simulink model "baroreflex"  (Simulink 6.6)
settings: Solver=ode45  StartTime=0.0  StopTime=100  RelTol=1e-3
undefined symbols (not defined in the file or in its folder): sigbuilder_block
settings Model: Creator=niumi  LastModifiedBy=mxkana
settings DebuggingCC: MultiTaskDSMMsg=warning  MultiTaskCondExecSysMsg=none  StrictBusMsg=None
settings RTWCC: IncludeERTFirstTime=on

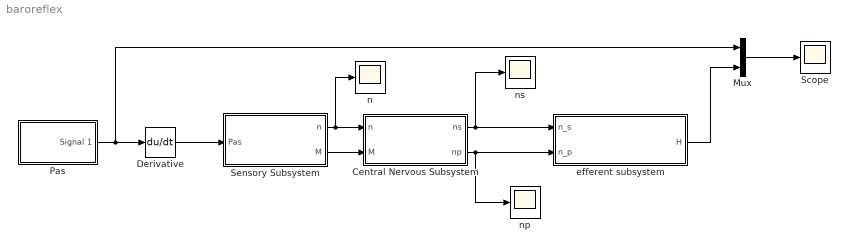
== system baroreflex ==
  Central Nervous Subsystem : Subsystem
  Derivative : Derivative
  Mux : Mux  Inputs=2
  Pas : Subsystem  Tag=STV Subsys  LoadFcn=sigbuilder_block('load');  StartFcn=sigbuilder_block('start');  StopFcn=sigbuilder_block('stop');  ClipboardFcn=sigbuilder_block('clipboard');  mask(Sigbuilder block){}
      mask help: Sigbuilder GUI
      mask init:
      | if ~strcmp(get_param(bdroot(gcbh),'SimulationStatus'),'stopped') tuvar = sigbuilder_block('maskInit'); end
      settings: CopyFcn=sigbuilder_block('copy');  DeleteFcn=sigbuilder_block('delete');  ModelCloseFcn=sigbuilder_block('modelClose');  PreSaveFcn=sigbuilder_block('preSave');  NameChangeFcn=sigbuilder_block('namechange');  OpenFcn=sigbuilder_block('open',[79.5 60.75 747 469.5 ]);  CloseFcn=sigbuilder_block('close');
      mask Display: plot(0,0,100,100,[10,10,40,40,10],[80,20,20,80,80],[40,10],[50,50], [40,27,10],[65,72,56],[40,25,25,10],[28,28,43,43]);
  Scope : Scope
      settings: YMin=0  YMax=100
  Sensory Subsystem : Subsystem
  "efferent subsystem " : Subsystem  TreatAsAtomicUnit=on
  n : Scope
      settings: YMin=0  YMax=100
  np : Scope
      settings: YMin=0  YMax=100  SaveName=ScopeData3
  ns : Scope
      settings: YMin=0  YMax=100  SaveName=ScopeData2
  wires:
  Sensory Subsystem/1(n) -> Central Nervous Subsystem/1(n), n/1
  Central Nervous Subsystem/1(ns) -> "efferent subsystem "/1(n_s), ns/1
  Central Nervous Subsystem/2(np) -> "efferent subsystem "/2(n_p), np/1
  Derivative/1 -> Sensory Subsystem/1(Pas)
  Pas/1(Signal 1) -> Derivative/1, Mux/1
  "efferent subsystem "/1(H) -> Mux/2
  Mux/1 -> Scope/1
  Sensory Subsystem/2(M) -> Central Nervous Subsystem/2(M)

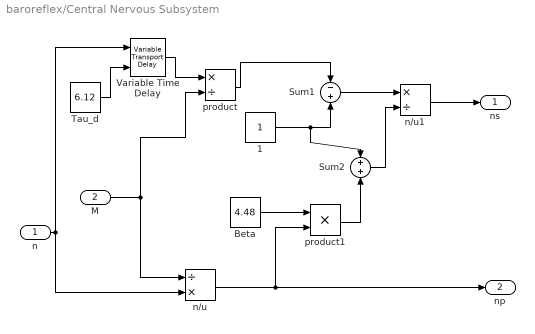
== system baroreflex/Central Nervous Subsystem ==
  n : Inport
  M : Inport  Port=2
  1 : Constant
  Beta : Constant  Value=4.48
  Sum1 : Sum  Inputs=-+
  Sum2 : Sum
  Tau_d : Constant  Value=6.12
  Variable Time Delay : VariableTransportDelay  MaximumDelay=10
  n/u : Product  Inputs=/*  OutScaling=2^-10
  n/u1 : Product  Inputs=*/  OutScaling=2^-10
  product : Product  Inputs=*/  OutScaling=2^-10
  product1 : Product  Inputs=**  OutScaling=2^-10
  ns : Outport
  np : Outport  Port=2
  wires:
  product/1 -> Sum1/1
  1/1 -> Sum1/2, Sum2/1
  n/1 -> Variable Time Delay/1, n/u/2
  n/u/1 -> np/1, product1/2
  Sum1/1 -> n/u1/1
  Sum2/1 -> n/u1/2
  n/u1/1 -> ns/1
  Tau_d/1 -> Variable Time Delay/2
  Variable Time Delay/1 -> product/1
  Beta/1 -> product1/1
  product1/1 -> Sum2/2
  M/1 -> n/u/1, product/2

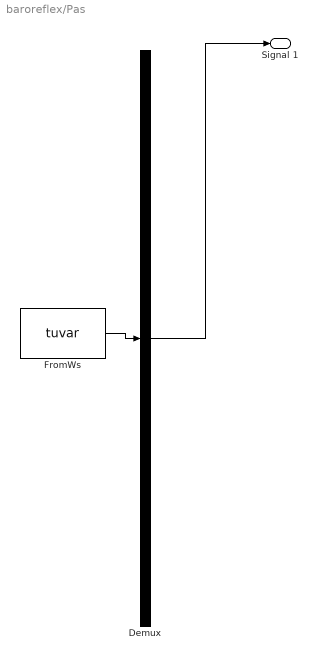
== system baroreflex/Pas ==
  Demux : Demux  Tag=STV Demux  Outputs=1
  FromWs : FromWorkspace  Tag=STV FromWs  VariableName=tuvar  SampleTime=0  SigBuilderData=DataTag0  VnvData=DataTag1
      SigBuilderData=|
      | channels.label = 'Signal 1'
      | channels.allXData = {[0 1.3 16.3 23.1 39 48.5 64.7 71.1 88.8 100]}
      | channels.allYData = {[90 85 150 110 149 60 65 80 180 110]}
      | common.afterFinalStr = 'Extrapolate'
      | common.sampleTime = 0
      | dataSet.timeRange = [0 100]
      | dataSet.name = 'Group 1'
  Signal 1 : Outport  Tag=STV Outport
  wires:
  Demux/1 -> Signal 1/1
  FromWs/1 -> Demux/1

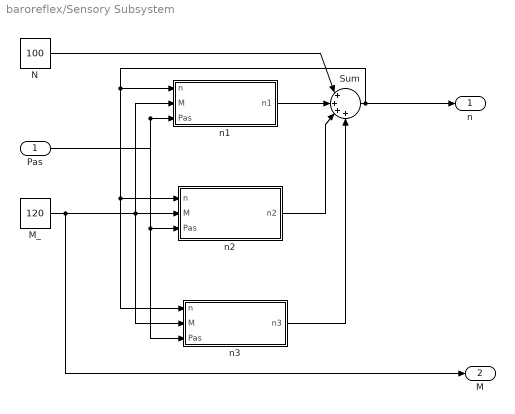
== system baroreflex/Sensory Subsystem ==
  Pas : Inport
  M_ : Constant  Value=120
  N : Constant  Value=100
  Sum : Sum  Inputs=|++++
  n1 : Subsystem
  n2 : Subsystem
  n3 : Subsystem
  n : Outport
  M : Outport  Port=2
  wires:
  n1/1(n1) -> Sum/2
  n2/1(n2) -> Sum/3
  Sum/1 -> n1/1(n), n2/1(n), n3/1(n), n/1
  M_/1 -> n1/2(M), n2/2(M), n3/2(M), M/1
  Pas/1 -> n1/3(Pas), n2/3(Pas), n3/3(Pas)
  N/1 -> Sum/1
  n3/1(n3) -> Sum/4

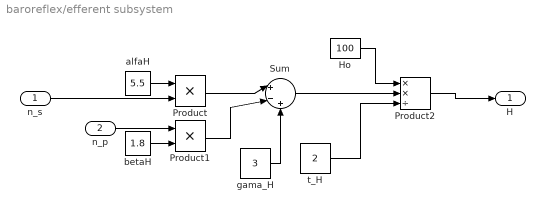
== system baroreflex/efferent subsystem  ==
  n_s : Inport
  n_p : Inport  Port=2
  Ho : Constant  Value=100
  Product : Product  RndMeth=Zero
  Product1 : Product  RndMeth=Zero
  Product2 : Product  Inputs=**/  RndMeth=Zero
  Sum : Sum  Inputs=|+-+
  alfaH : Constant  Value=5.5
  betaH : Constant  Value=1.8
  gama_H : Constant  Value=3
  t_H : Constant  Value=2
  H : Outport
  wires:
  alfaH/1 -> Product/1
  n_s/1 -> Product/2
  n_p/1 -> Product1/1
  betaH/1 -> Product1/2
  gama_H/1 -> Sum/3
  Product/1 -> Sum/1
  Product1/1 -> Sum/2
  t_H/1 -> Product2/3
  Sum/1 -> Product2/2
  Ho/1 -> Product2/1
  Product2/1 -> H/1

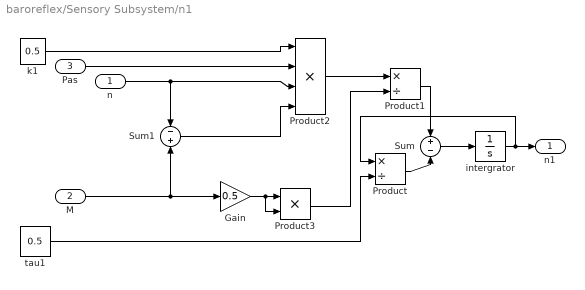
== system baroreflex/Sensory Subsystem/n1 ==
  n : Inport
  M : Inport  Port=2
  Pas : Inport  Port=3
  Gain : Gain  Gain=0.5
  Product : Product  Inputs=*/  RndMeth=Zero
  Product1 : Product  Inputs=*/  RndMeth=Zero
  Product2 : Product  Inputs=4  RndMeth=Zero
  Product3 : Product  RndMeth=Zero
  Sum : Sum  Inputs=+-
  Sum1 : Sum  Inputs=-+
  intergrator : Integrator
  k1 : Constant  Value=0.5
  tau1 : Constant  Value=0.5
  n1 : Outport
  wires:
  Product/1 -> Sum/2
  tau1/1 -> Product/2
  Product1/1 -> Sum/1
  Product2/1 -> Product1/1
  k1/1 -> Product2/1
  Pas/1 -> Product2/2
  n/1 -> Product2/3, Sum1/1
  Sum1/1 -> Product2/4
  M/1 -> Sum1/2, Gain/1
  Product3/1 -> Product1/2
  Gain/1 -> Product3/1, Product3/2
  Sum/1 -> intergrator/1
  intergrator/1 -> n1/1, Product/1

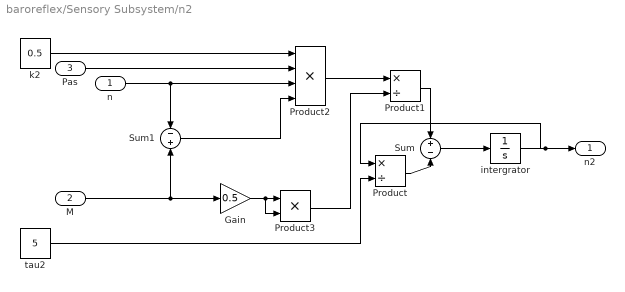
== system baroreflex/Sensory Subsystem/n2 ==
  n : Inport
  M : Inport  Port=2
  Pas : Inport  Port=3
  Gain : Gain  Gain=0.5
  Product : Product  Inputs=*/  RndMeth=Zero
  Product1 : Product  Inputs=*/  RndMeth=Zero
  Product2 : Product  Inputs=4  RndMeth=Zero
  Product3 : Product  RndMeth=Zero
  Sum : Sum  Inputs=+-
  Sum1 : Sum  Inputs=-+
  intergrator : Integrator
  k2 : Constant  Value=0.5
  tau2 : Constant  Value=5
  n2 : Outport
  wires:
  Product/1 -> Sum/2
  tau2/1 -> Product/2
  Product1/1 -> Sum/1
  Product2/1 -> Product1/1
  k2/1 -> Product2/1
  Pas/1 -> Product2/2
  n/1 -> Product2/3, Sum1/1
  Sum1/1 -> Product2/4
  M/1 -> Sum1/2, Gain/1
  Product3/1 -> Product1/2
  Gain/1 -> Product3/1, Product3/2
  Sum/1 -> intergrator/1
  intergrator/1 -> n2/1, Product/1

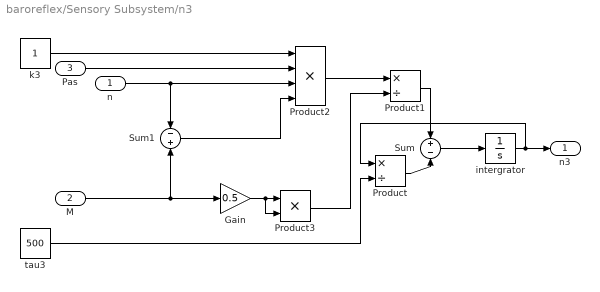
== system baroreflex/Sensory Subsystem/n3 ==
  n : Inport
  M : Inport  Port=2
  Pas : Inport  Port=3
  Gain : Gain  Gain=0.5
  Product : Product  Inputs=*/  RndMeth=Zero
  Product1 : Product  Inputs=*/  RndMeth=Zero
  Product2 : Product  Inputs=4  RndMeth=Zero
  Product3 : Product  RndMeth=Zero
  Sum : Sum  Inputs=+-
  Sum1 : Sum  Inputs=-+
  intergrator : Integrator
  k3 : Constant
  tau3 : Constant  Value=500
  n3 : Outport
  wires:
  Product/1 -> Sum/2
  tau3/1 -> Product/2
  Product1/1 -> Sum/1
  Product2/1 -> Product1/1
  k3/1 -> Product2/1
  Pas/1 -> Product2/2
  n/1 -> Product2/3, Sum1/1
  Sum1/1 -> Product2/4
  M/1 -> Sum1/2, Gain/1
  Product3/1 -> Product1/2
  Gain/1 -> Product3/1, Product3/2
  Sum/1 -> intergrator/1
  intergrator/1 -> n3/1, Product/1
